simulink model "MotorDCImaPermanente"  (R2018a)
settings: Solver=VariableStepAuto  StartTime=0.0  StopTime=10.0  RelTol=1e-3
undefined symbols (not defined in the file): J, Lc, Rc
libraries: powerlib x5, pePwmGenerator x1
settings Model: Creator=MATHEUS  LastModifiedBy=MATHEUS

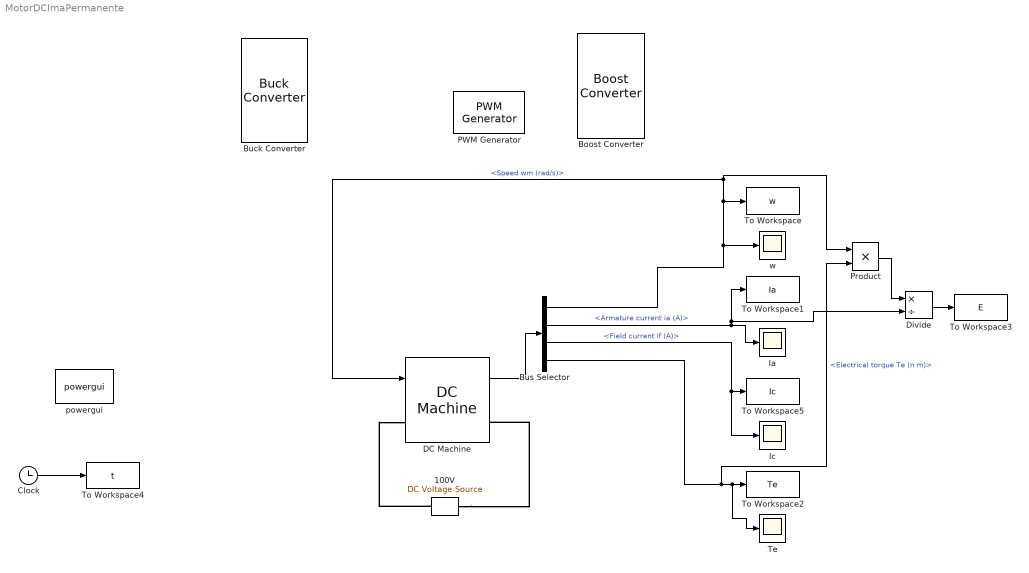
== system MotorDCImaPermanente ==
  100V : powerlib/Electrical Sources/DC Voltage Source  Amplitude=100  Measurements=None
  Boost Converter : powerlib/Power Electronics/Boost Converter  ModelType=Switching devices  Ron=1e-3  Rs=1e6  Cs=inf  Vforward=[0,0]  Ron_Diode=1e-3  Rs_Diode=1e6  Cs_Diode=inf  Vf_Diode=1e-3  Rs_CurrentSource=inf
      settings: SourceProductName=Simscape Power Systems  SourceProductBaseCode=PS
  Buck Converter : powerlib/Power Electronics/Buck Converter  ModelType=Switching devices  Ron=1e-3  Rs=1e6  Cs=inf  Vforward=[0,0]  Ron_Diode=1e-3  Rs_Diode=1e6  Cs_Diode=inf  Vf_Diode=1e-3  Rs_CurrentSource=inf
      settings: SourceProductName=Simscape Power Systems  SourceProductBaseCode=PS
  Bus Selector : BusSelector  OutputSignals=Speed wm (rad/s),Armature current ia (A),Field current if (A),Electrical torque Te (n m)
  Clock : Clock
  DC Machine : powerlib/Machines/DC Machine  PresetModel=No  MechanicalLoad=Speed w  FieldType=Permanent magnet  ShowDetailedParameters=on  MeasurementBus=on  RLa=[ 1 0.01]  RLf=[ Rc Lc ]  Laf=Lac  MachineConstant=Torque constant (N.m/A)  Ke=1.8  Kt=0  J=J  Bm=B  Tf=Tf  w0=W  Ifinit=Ic  TsPowergui=0  TsBlock=-1
  Divide : Product  Inputs=*/
  Ia : Scope
  Ic : Scope
  PWM Generator : pePwmGenerator/PWM Generator  CarrCount=Up  Tper=0.001  Ts=5e-5
  Product : Product
  Te : Scope
  To Workspace : ToWorkspace  VariableName=w  SampleTime=-1
  To Workspace1 : ToWorkspace  VariableName=Ia  SampleTime=-1
  To Workspace2 : ToWorkspace  VariableName=Te  SampleTime=-1
  To Workspace3 : ToWorkspace  VariableName=E  SampleTime=-1
  To Workspace4 : ToWorkspace  VariableName=t  SampleTime=-1
  To Workspace5 : ToWorkspace  VariableName=Ic  SampleTime=-1
  powergui : powerlib/powergui  Priority=1  SimulationMode=Continuous  SampleTime=50e-6  frequency=60  Iterations=50  frequencyindice=0  Pbase=100e6  ErrMax=1e-4  UnitsV=kV  UnitsW=MW  buscounter=0  FunctionMessages=off  echomessages=off  EnableUseOfTLC=off  CurrentSourceSwitches=off  DisableSnubberDevices=off  DisableRonSwitches=off  DisableVfSwitches=off  DisplayEquations=off  SolverType=Tustin/Backward Euler (TBE)  Interpol=off  ExternalGateDelay=off  methode=off  Ts=10  x0status=blocks  SPID=off  SwTol=0  HookPort=off  RestoreLinks=warning  ResistiveCurrentMeasurement=off  Frange=[0:2:500]  Ylog=off  Xlog=on  ShowGrid=off  save=off  variable=ZData  structure=0  ZoomFFT=off  StartTime=0.0  cycles=1  DisplayStyle=1  fundamental=60  FreqAxis=off  MaxFrequency=1000  frequencyindicesteady=1  RmsSteady=1  display=off
  w : Scope
  wires:
  Product/1 -> Divide/1
  Bus Selector/1 -> DC Machine/1, Product/1, To Workspace/1, w/1  "<Speed wm (rad/s)>"
  Bus Selector/3 -> Ic/1, To Workspace5/1  "<Field current if (A)>"
  Clock/1 -> To Workspace4/1
  Bus Selector/2 -> Ia/1, To Workspace1/1, Divide/2  "<Armature current ia (A)>"
  Bus Selector/4 -> Product/2, Te/1, To Workspace2/1  "<Electrical torque Te (n m)>"
  Divide/1 -> To Workspace3/1
  DC Machine/1 -> Bus Selector/1
  connections:
  100V/RConn1 -- DC Machine/LConn1
  100V/LConn1 -- DC Machine/RConn1
